simulink model "Test_Commande"  (R2020b)
settings: Solver=VariableStepAuto  StartTime=0.0  StopTime=10.0  RelTol=1e-3
undefined symbols (not defined in the file or in its folder): A, A_K1, B, B_K1, C, C_K1, D, D_K1
settings Model: Creator=Sandou  LastModifiedBy=Sandou

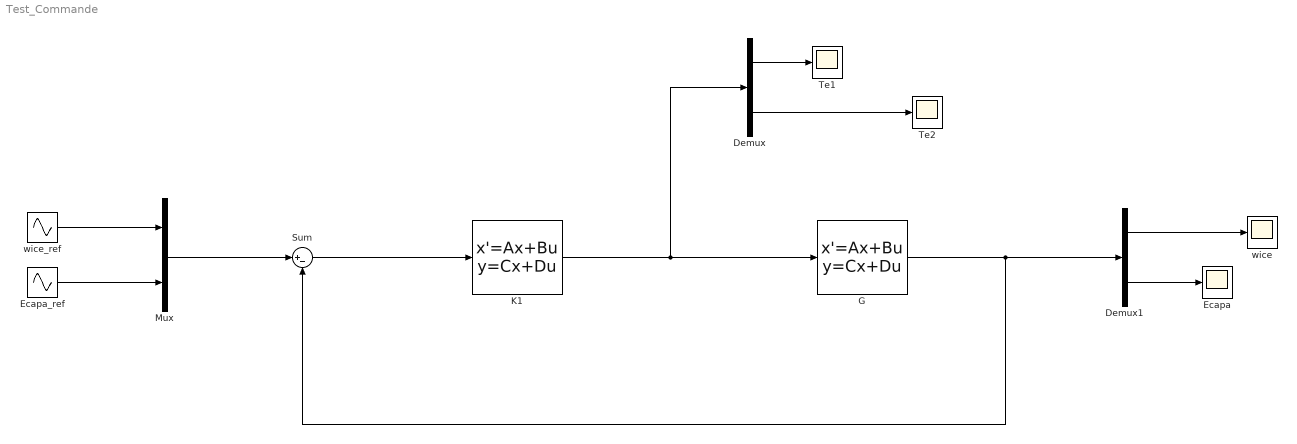
== system Test_Commande ==
  Demux : Demux  Outputs=2
  Demux1 : Demux  Outputs=2
  Ecapa : Scope
  Ecapa_ref : Sin  Amplitude=0  Frequency=40  Phase=-3.04  SampleTime=0
  G : StateSpace  A=A  B=B  C=C  D=D  InitialCondition=0
  K1 : StateSpace  A=A_K1  B=B_K1  C=C_K1  D=D_K1  InitialCondition=0
  Mux : Mux  Inputs=2
  Sum : Sum  Inputs=|+-
  Te1 : Scope
  Te2 : Scope
  wice : Scope
  wice_ref : Sin  Frequency=40  SampleTime=0
  wires:
  K1/1 -> Demux/1, G/1
  Sum/1 -> K1/1
  G/1 -> Demux1/1, Sum/2
  Mux/1 -> Sum/1
  Demux/1 -> Te1/1
  Demux/2 -> Te2/1
  wice_ref/1 -> Mux/1
  Ecapa_ref/1 -> Mux/2
  Demux1/1 -> wice/1
  Demux1/2 -> Ecapa/1
